simulink model "SMD_Laplace_Form"  (R2024b)
settings: Solver=VariableStepAuto  StartTime=0.0  StopTime=100  MaxStep=0.001  RelTol=1e-3
values from neighbouring files (symbols this model uses):
  b = 3.5077E-6    (= 3.5077e-06)    [DC_Motor_run.m]    (also in PID_Controlled_SPD_run.m = 10; run_SMD_Laplace.m = 0.1; run_Spring_mass_Damper.m = 10)
  F = 1    [PID_Controlled_SPD_run.m]    (also in closed_loop_code.m = 2; run_SMD_Laplace.m; run_Spring_mass_Damper.m = 10)
  k = 20    [PID_Controlled_SPD_run.m]    (also in run_SMD_Laplace.m; run_Spring_mass_Damper.m)
  M = 1    [PID_Controlled_SPD_run.m]    (also in run_SMD_Laplace.m; run_Spring_mass_Damper.m)
libraries: dspsrcs4 x1
settings Model: Creator=sajim  LastModifiedBy=sajim

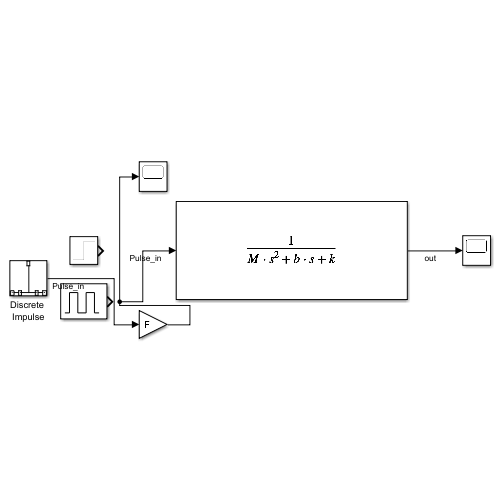
[thumbnail: Simulink's stored preview of the top-level diagram]
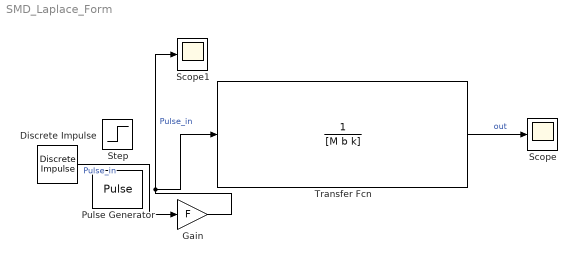
== system SMD_Laplace_Form ==
  Discrete Impulse : dspsrcs4/Discrete  Impulse  Delay=0  SampleTime=1  FrameSample=1  OutputFrames=off  dataType=double  isSigned=on  wordLen=16  udDataType=sfix(16)  fracBitsMode=Best precision  numFracBits=15  OutDataTypeStr=double  LastOutDataTypeStr=double
  Gain : Gain  Gain=F
  Pulse Generator : DiscretePulseGenerator  PulseType=Time based  Amplitude=F  Period=10  PulseWidth=5
  Scope : Scope
  Scope1 : Scope
  Step : Step  SampleTime=0
  Transfer Fcn : TransferFcn  Denominator=[M b k]
  wires:
  Transfer Fcn/1 -> Scope/1  "out"
  Gain/1 -> Scope1/1, Transfer Fcn/1  "Pulse_in"
  Discrete Impulse/1 -> Gain/1  "Pulse_in"
